simulink model "external_memory_test"  (R2020b)
settings: Solver=FixedStepDiscrete  StartTime=0.0  StopTime=80  RelTol=1e-3
InitFcn:
  | Feature_Width = 64;
  | Feature_Height = 64;
  | Weight_Width = 3;
  | Weight_Height = 3;
  | external_memory_test_init;
values from neighbouring files (symbols this model uses):
  Burst_Length = Feature_Weight_Length    [external_memory_test_init.m]
  byPass = 1    [external_memory_test_init.m]
  Conv_Padding = 0    [external_memory_test_init.m]
  Conv_Stride = 1    [external_memory_test_init.m]
  DDR_Depth = Weight_Length + Feature_Length + outFeature_Length    [external_memory_test_init.m]
  ddrInitData = single((rand(1,DDR_Depth)))    [external_memory_test_init.m]
  Duty_Cycle = 0.5    [external_memory_test_init.m]
  Feature_Area = Feature_Width * Feature_Height    [external_memory_test_init.m]
  Feature_Length = Phase_In * Feature_Area    [external_memory_test_init.m]
  inChannel = 3    [external_memory_test_init.m]
  outChannel = 2    [external_memory_test_init.m]
  outFeature_Length = outFeature_Width * outFeature_Height * Phase_Out    [external_memory_test_init.m]
  Pool_Stride = 2    [external_memory_test_init.m]
  Pool_Width = 2    [external_memory_test_init.m]
  Tc = 1    [external_memory_test_init.m]
  Ti = 1    [external_memory_test_init.m]
  To = 1    [external_memory_test_init.m]
  Tr = 1    [external_memory_test_init.m]
  Weight_Length = Phase_In * Weight_Area * Phase_Out    [external_memory_test_init.m]
undefined symbols (not defined in the file or in its folder): Conv_Step, Pool_Step, sigbuilder_block
libraries: hdlsllib x85, simulink x44, visionhdlutilities x16
(part 6 of 6)

== matlab function external_memory_test/DUT/2DConvPE V1.2/MATLAB Function ==
  settings: fimath=fimath('RoundingMethod', 'Floor','OverflowAction', 'Wrap','ProductMode', 'FullPrecision', 'SumMode', 'FullPrecision')
  data: w0 output; dataIn input; w1 output; rst input; write_en input; w2 output; w3 output; w4 output; w5 output; w6 output; w7 output; w8 output
function [w0, w1, w2, w3 , w4, w5, w6, w7, w8] = weight_register(dataIn, rst, write_en)
%#codegen
persistent read_cnt;

% Counter
if(isempty(read_cnt))
   read_cnt = fi(0,1,32,0); 
end

% Max Count = uint32(8)
persistent cntMax;

if(isempty(cntMax))
   cntMax = fi(9 - 1,1,32,0);
end

% weight0
persistent weight0
if(isempty(weight0))
   weight0 = fi(0,1,32,0); 
end

% weight1
persistent weight1
if(isempty(weight1))
   weight1 = fi(0,1,32,0); 
end

% weight2
persistent weight2
if(isempty(weight2))
   weight2 = fi(0,1,32,0); 
end

% weight3
persistent weight3
if(isempty(weight3))
   weight3 = fi(0,1,32,0); 
end

% weight1
persistent weight4
if(isempty(weight4))
   weight4 = fi(0,1,32,0); 
end

% weight5
persistent weight5
if(isempty(weight5))
   weight5 = fi(0,1,32,0); 
end

% weight6
persistent weight6
if(isempty(weight6))
   weight6 = fi(0,1,32,0); 
end

% weight7
persistent weight7
if(isempty(weight7))
   weight7 = fi(0,1,32,0); 
end

% weight8
persistent weight8
if(isempty(weight8))
   weight8 = fi(0,1,32,0); 
end

%%%%%%%%%%%%%%%%%%%%%%%%%%%%%%%%%%%%
% Output Logic
    w0 = weight0;
    w1 = weight1;
    w2 = weight2;
    w3 = weight3;
    w4 = weight4;
    w5 = weight5;
    w6 = weight6;
    w7 = weight7;
    w8 = weight8;
%%%%%%%%%%%%%%%%%%%%%%%%%%%%%%%%%%%%

if (rst == 1)
    % reset the output
    read_cnt = fi(0,1,32,0);
    
    weight0 = fi(0,1,32,0);
    weight1 = fi(0,1,32,0);
    weight2 = fi(0,1,32,0);
    weight3 = fi(0,1,32,0);
    weight4 = fi(0,1,32,0);
    weight5 = fi(0,1,32,0);
    weight6 = fi(0,1,32,0);
    weight7 = fi(0,1,32,0);
    weight8 = fi(0,1,32,0);
elseif (write_en == 1)
    if (read_cnt == cntMax)
        read_cnt = fi(0,1,32,0);
        weight0 = fi(dataIn,1,32,0);
    else
        if (read_cnt == 0)
           weight8 = fi(dataIn,1,32,0);
        elseif (read_cnt == 1)
            weight5 = fi(dataIn,1,32,0);
        elseif (read_cnt == 2)
            weight2 = fi(dataIn,1,32,0);
        elseif (read_cnt == 3)
            weight7 = fi(dataIn,1,32,0);
        elseif (read_cnt == 4)
            weight4 = fi(dataIn,1,32,0);
        elseif (read_cnt == 5)
            weight1 = fi(dataIn,1,32,0);
        elseif (read_cnt == 6)
            weight6 = fi(dataIn,1,32,0);
        elseif (read_cnt == 7)
            weight3 = fi(dataIn,1,32,0);
        end   
        read_cnt = fi(read_cnt+1, 1,32,0);
    end
end

== matlab function external_memory_test/DUT/2DConvPE V1.3/MATLAB Function ==
  settings: fimath=fimath('RoundingMethod', 'Floor','OverflowAction', 'Wrap','ProductMode', 'FullPrecision', 'SumMode', 'FullPrecision')
  data: w0 output; dataIn input; w1 output; rst input; write_en input; w2 output; w3 output; w4 output; w5 output; w6 output; w7 output; w8 output
function [w0, w1, w2, w3 , w4, w5, w6, w7, w8] = weight_register(dataIn, rst, write_en)
%#codegen
persistent read_cnt;

% Counter
if(isempty(read_cnt))
   read_cnt = fi(0,1,32,0); 
end

% Max Count = uint32(8)
persistent cntMax;

if(isempty(cntMax))
   cntMax = fi(9 - 1,1,32,0);
end

% weight0
persistent weight0
if(isempty(weight0))
   weight0 = fi(0,1,32,0); 
end

% weight1
persistent weight1
if(isempty(weight1))
   weight1 = fi(0,1,32,0); 
end

% weight2
persistent weight2
if(isempty(weight2))
   weight2 = fi(0,1,32,0); 
end

% weight3
persistent weight3
if(isempty(weight3))
   weight3 = fi(0,1,32,0); 
end

% weight1
persistent weight4
if(isempty(weight4))
   weight4 = fi(0,1,32,0); 
end

% weight5
persistent weight5
if(isempty(weight5))
   weight5 = fi(0,1,32,0); 
end

% weight6
persistent weight6
if(isempty(weight6))
   weight6 = fi(0,1,32,0); 
end

% weight7
persistent weight7
if(isempty(weight7))
   weight7 = fi(0,1,32,0); 
end

% weight8
persistent weight8
if(isempty(weight8))
   weight8 = fi(0,1,32,0); 
end

%%%%%%%%%%%%%%%%%%%%%%%%%%%%%%%%%%%%
% Output Logic
    w0 = weight0;
    w1 = weight1;
    w2 = weight2;
    w3 = weight3;
    w4 = weight4;
    w5 = weight5;
    w6 = weight6;
    w7 = weight7;
    w8 = weight8;
%%%%%%%%%%%%%%%%%%%%%%%%%%%%%%%%%%%%

if (rst == 1)
    % reset the output
    read_cnt = fi(0,1,32,0);
    
    weight0 = fi(0,1,32,0);
    weight1 = fi(0,1,32,0);
    weight2 = fi(0,1,32,0);
    weight3 = fi(0,1,32,0);
    weight4 = fi(0,1,32,0);
    weight5 = fi(0,1,32,0);
    weight6 = fi(0,1,32,0);
    weight7 = fi(0,1,32,0);
    weight8 = fi(0,1,32,0);
elseif (write_en == 1)
    if (read_cnt == cntMax)
        read_cnt = fi(0,1,32,0);
        weight0 = fi(dataIn,1,32,0);
    else
        if (read_cnt == 0)
           weight8 = fi(dataIn,1,32,0);
        elseif (read_cnt == 1)
            weight5 = fi(dataIn,1,32,0);
        elseif (read_cnt == 2)
            weight2 = fi(dataIn,1,32,0);
        elseif (read_cnt == 3)
            weight7 = fi(dataIn,1,32,0);
        elseif (read_cnt == 4)
            weight4 = fi(dataIn,1,32,0);
        elseif (read_cnt == 5)
            weight1 = fi(dataIn,1,32,0);
        elseif (read_cnt == 6)
            weight6 = fi(dataIn,1,32,0);
        elseif (read_cnt == 7)
            weight3 = fi(dataIn,1,32,0);
        end   
        read_cnt = fi(read_cnt+1, 1,32,0);
    end
end

== matlab function external_memory_test/DUT/DDR_Access/DDR Write Conroller ==
  settings: fimath=fimath('RoundingMethod', 'Floor','OverflowAction', 'Wrap','ProductMode', 'FullPrecision', 'SumMode', 'FullPrecision')
  data: ram_addr output; ddr_write_done output; burst_len input; start input boolean; wr_ready input; wr_addr output; wr_len output; wr_valid output; wr_complete input
function [ram_addr, ddr_write_done, wr_addr, wr_len, wr_valid] = fcn(burst_len, start, wr_ready, wr_complete)

[ram_addr, ddr_write_done, wr_addr, wr_len, wr_valid] = hdlcoder_external_memory_write_ctrl(burst_len, start, wr_ready, wr_complete);

end

== matlab function external_memory_test/DDR/load_init_data ==
  data: load_done output; ram_wr_data output; axi_wr_data input; axi_wr_add input; axi_wr_val input; ram_wr_add output; ram_wr_enb output boolean; INIT_ADDR parameter; DDR3_DEPTH parameter; INIT_DDR3 parameter; INIT_DATA parameter
function [load_done,ram_wr_data,ram_wr_add,ram_wr_enb] = load_init(axi_wr_data,axi_wr_add,axi_wr_val, INIT_ADDR, DDR3_DEPTH, INIT_DDR3,INIT_DATA)

%%%%%%%%%%%%%%%%%%%%%%%%%%%%%%%%%%%%%%%%%%%%%%%%%%%%%%
% Create persistent variables (registers)
persistent reg_ram_wr_add;
if(isempty(reg_ram_wr_add))
    reg_ram_wr_add = fi(0,0,32,0);
end

persistent reg_ram_wr_data;
if(isempty(reg_ram_wr_data))
    reg_ram_wr_data =cast(0,'like',axi_wr_data);% fi(0,1,ddrWidth,0);
end

persistent reg_ram_wr_data_d1;
if(isempty(reg_ram_wr_data_d1))
    reg_ram_wr_data_d1 = cast(0,'like',axi_wr_data);%
end


persistent state;
if(isempty(state))
    state = fi(0, 0, 3, 0);
end


persistent reg_ram_wr_enb;
if(isempty(reg_ram_wr_enb))
    reg_ram_wr_enb = false;
end

persistent reg_ram_wr_enb_d1;
if(isempty(reg_ram_wr_enb_d1))
    reg_ram_wr_enb_d1 = false;
end

persistent reg_init_data;
if(isempty(reg_init_data))
    reg_init_data = cast(zeros(1,DDR3_DEPTH),'like',axi_wr_data);% fi(zeros(1,DDR3_DEPTH),1,ddrWidth,0);
end

%%%%%%%%%%%%%%%%%%%%%%%%%%%%%%%%%%%%%%%%%%%%%%%%%%
% State Memory Encoding
INIT_ST    = fi(0, 0, 3, 0);
LOAD_START = fi(1, 0, 3, 0);
LOAD_PROG  = fi(3, 0, 3, 0);
LOAD_DONE  = fi(2, 0, 3, 0);
DATA_ST    = fi(6, 0, 3, 0);


% init phase states
% 1. Every state MUST assign every output value
% 2. Use explicit data type always
switch (state)
    case INIT_ST
       
        reg_ram_wr_add = fi(0,0,32,0);%uint32(0);
        reg_ram_wr_data =  cast(0,'like',axi_wr_data);%fi(0,1,ddrWidth,0);%int32(0);
        reg_ram_wr_enb = false;
        load_done = false;
        
    case LOAD_START
        
        reg_ram_wr_add = fi(INIT_ADDR,0,32,0);
        reg_ram_wr_data =  cast(reg_init_data(1,reg_ram_wr_add+1),'like',axi_wr_data);%fi(reg_init_data(1,reg_ram_wr_add+1),1,ddrWidth,0);%int32(INIT_DATA);
        reg_ram_wr_enb = true;
        load_done = false;
    case LOAD_PROG
        
        
        reg_ram_wr_add = fi(reg_ram_wr_add+1,0,32,0);
        reg_ram_wr_data =  cast(reg_init_data(1,reg_ram_wr_add+1),'like',axi_wr_data);%fi(reg_init_data(1,reg_ram_wr_add+1),1,ddrWidth,0);%int32(INIT_DATA);
        reg_ram_wr_enb = true;
        load_done = false;
    case LOAD_DONE
      
        reg_ram_wr_add = fi(reg_ram_wr_add,0,32,0);
       % reg_ram_wr_data = reg_ram_wr_data;%fi(reg_ram_wr_data,1,ddrWidth,0);
        reg_ram_wr_enb = true;
        load_done = true;
    case DATA_ST    
        %external (AXI ) inputs
        reg_ram_wr_add = fi(axi_wr_add,0,32,0);
        reg_ram_wr_data =  axi_wr_data;%fi(axi_wr_data,1,ddrWidth,0);
        reg_ram_wr_enb = axi_wr_val;
        load_done = true;
    otherwise
        
        reg_ram_wr_add = fi(0,0,32,0);
        reg_ram_wr_data =  cast(0,'like',axi_wr_data);%fi(0,1,ddrWidth,0);
        reg_ram_wr_enb = false;
        load_done = false;
end

ram_wr_add = fi(reg_ram_wr_add,0,32,0);
%ram_wr_data = reg_ram_wr_data;

if(load_done == true)
   ram_wr_data = cast(reg_ram_wr_data_d1,'like',axi_wr_data);%fi(reg_ram_wr_data_d1,1,ddrWidth,0);%reg_ram_wr_data_d1;
else
   ram_wr_data = cast(reg_ram_wr_data_d1,'like',axi_wr_data);%fi(reg_ram_wr_data_d1,1,ddrWidth,0);%reg_ram_wr_data;   
end


if(load_done == true)
   ram_wr_enb = reg_ram_wr_enb_d1;
else
   ram_wr_enb = reg_ram_wr_enb;   
end


if(load_done == false)
   reg_init_data = cast(INIT_DATA,'like',axi_wr_data);%fi(INIT_DATA,1,ddrWidth,0);%reg_ram_wr_data;   
end

reg_ram_wr_enb_d1 = reg_ram_wr_enb;
reg_ram_wr_data_d1 = reg_ram_wr_data;%fi(reg_ram_wr_data,1,ddrWidth,0);%int32(reg_ram_wr_data);
% Next State Logic
switch (state)
    case INIT_ST
        
        if ( INIT_DDR3 == true)
            nextState = LOAD_START;
        else
            nextState = DATA_ST;
        end
    case LOAD_START
            nextState = LOAD_PROG;
    case LOAD_PROG
        if(fi(ram_wr_add,0,32,0)==fi(DDR3_DEPTH-1,0,32,0))
            nextState = LOAD_DONE;
        else
            nextState = LOAD_PROG;
        end
    case LOAD_DONE
            nextState = DATA_ST;
    case DATA_ST
            nextState = DATA_ST; 
    otherwise
        nextState = INIT_ST;
end

state = nextState;

end

== matlab function external_memory_test/DDR/wrLogic/Wr_control/MATLAB Function ==
  data: axi_wr_en input; wr_leng output; axi_wr_length input; wr_ack input
function wr_leng = addr_latch(axi_wr_en,axi_wr_length,wr_ack)
%#codegen

persistent axi_wr_en_d1;
if(isempty(axi_wr_en_d1))
axi_wr_en_d1 = false;
end

persistent reg_len;
if(isempty(reg_len))
    reg_len = fi(0,0,32,0);%uint32(0);
end


persistent reg_len_d1;
if(isempty(reg_len_d1))
    reg_len_d1 = fi(0,0,32,0);%uint32(0);
end

reg_len_d1 = reg_len;
wr_leng = reg_len;

if((axi_wr_en==true)&&(axi_wr_en_d1==false)&&(reg_len_d1==0)) 
  reg_len= fi(axi_wr_length,0,32,0);%axi_wr_length;
elseif(wr_ack)
  reg_len= fi(0,0,32,0);%uint32(0);    
end

axi_wr_en_d1 = axi_wr_en;

== matlab function external_memory_test/DDR/rdLogic/rd_control ==
  data: axi_rd_add input; axi_rd_len input; axi_rd_val input; axi_rd_ready input; ram_rd_addr output; ram_rd_val output boolean; toggle parameter
function [ram_rd_addr, ram_rd_val] = rd_add_gen(axi_rd_add,axi_rd_len, axi_rd_val,axi_rd_ready,toggle)

%%%%%%%%%%%%%%%%%%%%%%%%%%%%%%%%%%%%%%%%%%%%%%%%%%%%%%
%%%Reg declaration
%RAM address generation counter
persistent ram_rd_cnt;

if(isempty(ram_rd_cnt))
    ram_rd_cnt = fi(0,0,32,0);%uint32(0);
end

%read response ack
persistent reg_rd_ack;

if(isempty(reg_rd_ack))
    reg_rd_ack = false;
end

%read status
persistent rd_progress;

if(isempty(rd_progress))
    rd_progress = false;
end

%read addr valid flag 
persistent rd_addr_val;

if(isempty(rd_addr_val))
    rd_addr_val = false;
end

%read addr valid flag 
persistent rd_addr_val_toggle;

if(isempty(rd_addr_val_toggle))
    rd_addr_val_toggle = false;
end

%start address and length of read burst latch
persistent start_addr;
if(isempty(start_addr))
    start_addr = fi(0,0,32,0);
end

persistent leng_latch;
if(isempty(leng_latch))
    leng_latch = fi(1,0,32,0);
end

%%%%%%%%%%%%%%%%%%%%%%%%%%%%%%%%%%%%%%%%%%%%%%%
%output
ram_rd_addr = (ram_rd_cnt);
ram_rd_val = (rd_addr_val);
%%%%%%%%%%%%%%%%%%%%%%%%%%%%%%%%%%%%%%%%%%%%%%%
if((reg_rd_ack == true)&&(axi_rd_ready == true))
    ram_rd_cnt = fi(start_addr,0,32,0);%uint32(start_addr );
    rd_addr_val = true;
elseif((rd_progress == true)&&(axi_rd_ready == true))
    
    if(rd_addr_val_toggle == true)
       ram_rd_cnt = fi(ram_rd_cnt + 1,0,32,0);%uint32(ram_rd_cnt + 1);
       rd_addr_val = true;
    else
       rd_addr_val = false;
   
    end
    if(toggle)
       rd_addr_val_toggle = ~(rd_addr_val_toggle);
    else
       rd_addr_val_toggle = true;
    end
elseif((rd_progress == false))  
    ram_rd_cnt = fi(0,0,32,0);%uint32(0) ;
    rd_addr_val = false;
else
    rd_addr_val = false;
end


%read progress flag
if((reg_rd_ack)&&(fi(ram_rd_cnt-start_addr,0,32,0)<fi(leng_latch-1,0,32,0)))
    rd_progress = true;
elseif(fi(ram_rd_cnt-start_addr,0,32,0)==fi(leng_latch-1,0,32,0))
    rd_progress = false;
end


%start address , length of burst latching
if(axi_rd_val)
    leng_latch(:) = axi_rd_len;
    start_addr(:) = axi_rd_add/4;
    reg_rd_ack = true;
else
    reg_rd_ack = false;
end

== matlab function external_memory_test/DUT/DDR_Access/DDR Read Conroller ==
  settings: fimath=fimath('RoundingMethod', 'Floor','OverflowAction', 'Wrap','ProductMode', 'FullPrecision', 'SumMode', 'FullPrecision')
  data: valid_out output; count_out output; ddr_read_done output; burst_len input; start input boolean; rd_aready input; rd_dvalid input; rd_addr output; rd_len output; rd_avalid output
function [valid_out, count_out, ddr_read_done, rd_addr, rd_len, rd_avalid] = fcn(burst_len, start, rd_aready, rd_dvalid)

[valid_out, count_out, ddr_read_done, rd_addr, rd_len, rd_avalid] = hdlcoder_external_memory_read_ctrl(burst_len, start, rd_aready, rd_dvalid);

end

== matlab function external_memory_test/DUT/2DConvPE V1.0/MATLAB Function ==
  settings: fimath=fimath('RoundingMethod', 'Floor','OverflowAction', 'Wrap','ProductMode', 'FullPrecision', 'SumMode', 'FullPrecision')
  data: w0 output; dataIn input; w1 output; rst input; write_en input; w2 output; w3 output; w4 output; w5 output; w6 output; w7 output; w8 output
function [w0, w1, w2, w3 , w4, w5, w6, w7, w8] = weight_register(dataIn, rst, write_en)
%#codegen
persistent read_cnt;

% Counter
if(isempty(read_cnt))
   read_cnt = fi(0,1,32,0); 
end

% Max Count = uint32(8)
persistent cntMax;

if(isempty(cntMax))
   cntMax = fi(9 - 1,1,32,0);
end

% weight0
persistent weight0
if(isempty(weight0))
   weight0 = fi(0,1,32,0); 
end

% weight1
persistent weight1
if(isempty(weight1))
   weight1 = fi(0,1,32,0); 
end

% weight2
persistent weight2
if(isempty(weight2))
   weight2 = fi(0,1,32,0); 
end

% weight3
persistent weight3
if(isempty(weight3))
   weight3 = fi(0,1,32,0); 
end

% weight1
persistent weight4
if(isempty(weight4))
   weight4 = fi(0,1,32,0); 
end

% weight5
persistent weight5
if(isempty(weight5))
   weight5 = fi(0,1,32,0); 
end

% weight6
persistent weight6
if(isempty(weight6))
   weight6 = fi(0,1,32,0); 
end

% weight7
persistent weight7
if(isempty(weight7))
   weight7 = fi(0,1,32,0); 
end

% weight8
persistent weight8
if(isempty(weight8))
   weight8 = fi(0,1,32,0); 
end

%%%%%%%%%%%%%%%%%%%%%%%%%%%%%%%%%%%%
% Output Logic
    w0 = weight0;
    w1 = weight1;
    w2 = weight2;
    w3 = weight3;
    w4 = weight4;
    w5 = weight5;
    w6 = weight6;
    w7 = weight7;
    w8 = weight8;
%%%%%%%%%%%%%%%%%%%%%%%%%%%%%%%%%%%%

if (rst == 1)
    % reset the output
    read_cnt = fi(0,1,32,0);
    
    weight0 = fi(0,1,32,0);
    weight1 = fi(0,1,32,0);
    weight2 = fi(0,1,32,0);
    weight3 = fi(0,1,32,0);
    weight4 = fi(0,1,32,0);
    weight5 = fi(0,1,32,0);
    weight6 = fi(0,1,32,0);
    weight7 = fi(0,1,32,0);
    weight8 = fi(0,1,32,0);
elseif (write_en == 1)
    if (read_cnt == cntMax)
        read_cnt = fi(0,1,32,0);
        weight0 = fi(dataIn,1,32,0);
    else
        if (read_cnt == 0)
           weight8 = fi(dataIn,1,32,0);
        elseif (read_cnt == 1)
            weight5 = fi(dataIn,1,32,0);
        elseif (read_cnt == 2)
            weight2 = fi(dataIn,1,32,0);
        elseif (read_cnt == 3)
            weight7 = fi(dataIn,1,32,0);
        elseif (read_cnt == 4)
            weight4 = fi(dataIn,1,32,0);
        elseif (read_cnt == 5)
            weight1 = fi(dataIn,1,32,0);
        elseif (read_cnt == 6)
            weight6 = fi(dataIn,1,32,0);
        elseif (read_cnt == 7)
            weight3 = fi(dataIn,1,32,0);
        end   
        read_cnt = fi(read_cnt+1, 1,32,0);
    end
end
